simulink model "euler1"  (R2025a)
settings: Solver=VariableStepAuto  StartTime=0.0  StopTime=10.0  RelTol=1e-3
values from neighbouring files (symbols this model uses):
  h = 0.1    [ejemplo_NOlineal_RK4.m]    (also in euler_explicita.m = (tf - t0)/n; euler_explicito.m = (tf - t0)/n; euler_midpoint.m = (tf - t0)/n; examplecrk4.m)
  y0 = 1    [ExampleEuler.m]    (also in ejemplo_NOlineal_RK4.m; examplecrk4.m; exmapleEuler2.m; lineal_RK4.m)
settings Model: Creator=a.diteodoro  LastModifiedBy=a.diteodoro

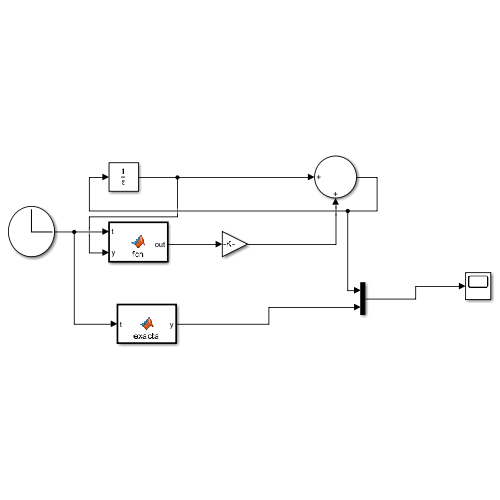
[thumbnail: Simulink's stored preview of the top-level diagram]
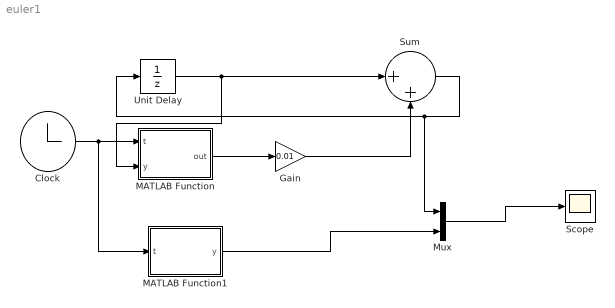
== system euler1 ==
  Clock : Clock
  Gain : Gain  Gain=0.01
  MATLAB Function : MATLAB Function  TreatAsAtomicUnit=on
  MATLAB Function1 : MATLAB Function  TreatAsAtomicUnit=on
  Mux : Mux  Inputs=2
  Scope : Scope
      settings: ActiveDisplayYMinimum=-0.14627505482983422  ActiveDisplayYMaximum=5.2995861194940215
  Sum : Sum  Inputs=|++
  Unit Delay : UnitDelay  InitialCondition=y0  SampleTime=h  HasFrameUpgradeWarning=on
  wires:
  Clock/1 -> MATLAB Function1/1(t), MATLAB Function/1(t)
  MATLAB Function/1(out) -> Gain/1
  Unit Delay/1 -> MATLAB Function/2(y), Sum/1
  Gain/1 -> Sum/2
  Sum/1 -> Mux/1, Unit Delay/1
  MATLAB Function1/1(y) -> Mux/2
  Mux/1 -> Scope/1

== matlab function euler1/MATLAB Function ==
  data: t input; out output; y input
function out = fcn(t, y)

out = -2*y + t;   % ejemplo
%out = y
end

== matlab function euler1/MATLAB Function1 ==
  data: t input; y output
function y = exacta(t)

y = 0.5*t - 0.25 + 1.25*exp(-2*t);

end
